simulink library "DigitalControlLib2"  (R2017b)
settings: Solver=VariableStepAuto  StartTime=0.0  StopTime=10.0  RelTol=1e-3
settings Model: Creator=alexandersoussan  LastModifiedBy=alexandersoussan

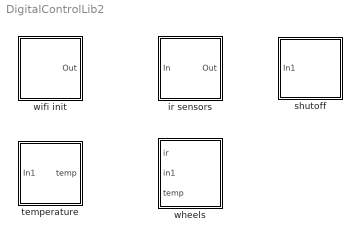
== system DigitalControlLib2 ==
  ir sensors : Subsystem
  shutoff : Subsystem
  temperature : Subsystem
  wheels : Subsystem
  wifi init : Subsystem

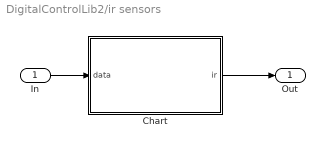
== system DigitalControlLib2/ir sensors ==
  In : Inport
  Chart : Stateflow chart  TreatAsAtomicUnit=on
  Out : Outport
  wires:
  In/1 -> Chart/1(data)
  Chart/1(ir) -> Out/1

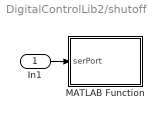
== system DigitalControlLib2/shutoff ==
  In1 : Inport
  MATLAB Function : MATLAB Function  TreatAsAtomicUnit=on
  wires:
  In1/1 -> MATLAB Function/1(serPort)

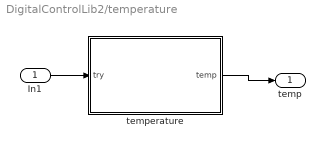
== system DigitalControlLib2/temperature ==
  In1 : Inport
  temperature : Stateflow chart  TreatAsAtomicUnit=on
  temp : Outport
  wires:
  temperature/1(temp) -> temp/1
  In1/1 -> temperature/1(try)

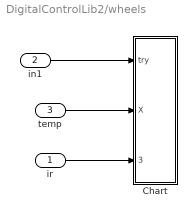
== system DigitalControlLib2/wheels ==
  ir : Inport
  in1 : Inport  Port=2
  temp : Inport  Port=3
  Chart : Stateflow chart  TreatAsAtomicUnit=on
  wires:
  ir/1 -> Chart/3(input1)
  temp/1 -> Chart/2(X)
  in1/1 -> Chart/1(try)

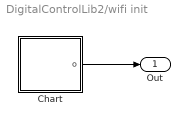
== system DigitalControlLib2/wifi init ==
  Chart : Stateflow chart  TreatAsAtomicUnit=on
  Out : Outport
  wires:
  Chart/1(o) -> Out/1

== stateflow chart DigitalControlLib2/temperature/temperature ==
  state temp
    en,du:
    temp=T;
  (default) -> temp
  data: y function_output; try input; temp output
  function y=T:
    | function y=T
    | persistent so
    | y=1;
    | coder.extrinsic('evalin');
    | coder.extrinsic('get');
    | 
    | so = evalin('base','objWs');
    | 
    | temp=0;  
    | coder.extrinsic('TemperatureRoomba');
    | temp=TemperatureRoomba(so);
    | 
    | y=temp;

== stateflow chart DigitalControlLib2/ir sensors/Chart ==
  state RANGE
    en,du:
    ir=irv;
  (default) -> RANGE
  data: y function_output; data input; ir output
  function y = irv:
    | function y = irv
    | y = [0,0,0,0,0,0];
    | persistent obj
    | coder.extrinsic('evalin')
    | coder.extrinsic('get')
    | coder.extrinsic('RangeStateRoomba')
    | if isempty(obj)
    |     obj = evalin('base','objWs')
    | end
    | coder.extrinsic('RangeStateRoomba')
    | y = RangeStateRoomba(obj);

== stateflow chart DigitalControlLib2/wifi init/Chart ==
  state INIT
    en,du:
    tcpInit;
    o=1;
  (default) -> INIT
  data: o output
  function tcpInit:
    | function tcpInit
    | coder.extrinsic('RoombaWifiInit');
    | coder.extrinsic('assignin');
    | persistent obj
    | if isempty(obj)
    | obj = RoombaWifiInit('10.0.0.1','full');
    | assignin('base','objWs', obj);
    | end

== matlab function DigitalControlLib2/shutoff/MATLAB Function ==
  data: serPort input
function PowerOffRoomba(serPort)
% PowerOffRoomba(serPort)
% Power down robot.  
% serPort is a serial port object created by RoombaInit
% Note that the physical power button does not work, and power saving and charging will not
% occur once the robot is initialized with RoombaInit.  There is a real
% risk of deeply discharging the Roomba's battery causing permanent
% damage.  Always use this command when done! 
% By Joel Esposito, US Naval Academy 2015
fwrite(serPort, [141 3]); % play RoombaInit song
pause(1);
fwrite(serPort, 133);

== stateflow chart DigitalControlLib2/wheels/Chart ==
  state on1
    state off
      en,du:
      wheel(0,0);
    state on
      state Reverse
        entry:
        wheel(-.1,-0.1);
      state Straiforward
        entry,du:
        wheel(0.05,0.05);
      state Rightturn3
        entry,du:
        wheel(-0.2,0.2);
      state leftturn3
        entry,du:
        wheel(0.2,-0.2);
      state Leftturn3
        entry,du:
        wheel(0.3,-0.2);
      state Rightturn2
        entry,du:
        wheel(-0.2,0.3);
      state Leftturn2
        entry,du:
        wheel(0.2,-0.1);
      state Rightturn1
        entry,du:
        wheel(-0.1,.2);
      (default) -> Reverse
      Reverse -> Straiforward : after(1,sec)
      Straiforward -> Rightturn1 [order 1] : [input1(1)>0]
      Rightturn1 -> Straiforward : [input1(1)<1]
      Straiforward -> Rightturn2 [order 2] : [input1(2)>0]
      Rightturn2 -> Straiforward : [input1(2)<1]
      Straiforward -> Rightturn3 [order 3] : [input1(3)>0]
      Rightturn3 -> Straiforward : [input1(3)<1]
      Straiforward -> leftturn3 [order 4] : [input1(4)>0]
      leftturn3 -> Straiforward : [input1(4)<1]
      Straiforward -> Leftturn3 [order 5] : [input1(5)>0]
      Leftturn3 -> Straiforward : [input1(5)<1]
      Straiforward -> Leftturn2 [order 6] : [input1(6)>0]
      Leftturn2 -> Straiforward : [input1(6)<1]
    (default) -> off
    off -> on : [X<80]
    on -> off : [X>=80]
  (default) -> on1
  data: u1 function_input; u2 function_input; try input; X input; input1 input
  function wheel(u1,u2):
    | function wheel(u1,u2)
    | persistent so
    | coder.extrinsic('evalin');
    | coder.extrinsic('get');
    | so = evalin('base','objWs');
    | coder.extrinsic('SetWheelVelRoomba');
    | SetWheelVelRoomba(so,u1 , u2);
